simulink model "HydroPowertest"  (R2024b)
settings: Solver=FixedStepAuto  StartTime=0.0  StopTime=10  FixedStep=0.0001  RelTol=1e-3
values from neighbouring files (symbols this model uses):
  A = [0 Lq 0;-Ld 0 Mf]    [Generator_Datatest.m]
  Acc = [0 Lq 0;-Ld 0 Mf;0 0 0]    [Generator_Datatest.m]
  Af = 0.01    [Data__MOTOR.m]    (also in Generator_Data.m = 0.0001; Generator_Datatest.m)
  Bf = 0.0002    [Data__MOTOR.m]    (also in Generator_Data.m = 2e-05; Generator_Datatest.m)
  Cc = Cc0+6*Cc0    (= 0.7)    [Data__MOTOR.m]    (also in Generator_Datatest.m)
  Cc0 = 0.1    [Data__MOTOR.m]    (also in Generator_Datatest.m)
  CurrentFaultSwitch = 0    [Data__MOTOR.m]    (also in Generator_Data.m = 1; Generator_Datatest.m)
  Jm = 0.08    [Data__MOTOR.m]    (also in Generator_Datatest.m)
  Ke = 0.139    [Data__MOTOR.m]    (also in Generator_Datatest.m)
  Lcc = [-Ld 0 Mf;0 -Lq 0;-Mf 0 Lf]    [Generator_Datatest.m]
  Le = 0.44    [Data__MOTOR.m]    (also in Generator_Datatest.m)
  Lf = 0.0924    [Generator_Datatest.m]
  P = 4    [Generator_Data.m]    (also in Generator_Datatest.m = 3)
  R = 42.3    [Data__MOTOR.m]    (also in Generator_Datatest.m = [Rs 0 0;0 Rs 0])
  rate_noise_i = 0.02*In    (= 0.22)    [Data__MOTOR.m]    (also in Generator_Data.m = 0.02; Generator_Datatest.m)
  rate_noise_w = 0.02*Wn    (= 2.96)    [Data__MOTOR.m]    (also in Generator_Data.m = 0.002; Generator_Datatest.m)
  Rcc = [Rs 0 0;0 Rs 0;0 0 Rf]    [Generator_Datatest.m]
  Re = 2.4    [Data__MOTOR.m]    (also in Generator_Datatest.m)
  Rf = 10    [Generator_Datatest.m]
  Rm = 0.01    [Data__MOTOR.m]    (also in Generator_Datatest.m)
  sinamp = 384.6    [Generator_Datatest.m]
  StartStop = 0    [Data__MOTOR.m]    (also in Generator_Data.m; Generator_Datatest.m)
  Te = 0.1    [Data__MOTOR.m]    (also in Generator_Data.m = 1; Generator_Datatest.m)
  Ua = 48    [Data__MOTOR.m]    (also in Generator_Datatest.m)
  VelocityFaultSwitch = 0    [Data__MOTOR.m]    (also in Generator_Data.m = 1; Generator_Datatest.m)
  Vf = 300    [Generator_Datatest.m]
undefined symbols (not defined in the file or in its folder): dspblkCoreblockFVToolHelper, gcbh, sigbuilder_block
libraries: SignalEditorBlockLib x5
(part 1 of 3)
settings Model: Creator=belka  LastModifiedBy=Nasser
settings DebuggingCC: SignalResolutionControl=TryResolveAll
settings RTWCC: GPUComputeCapability=3.5

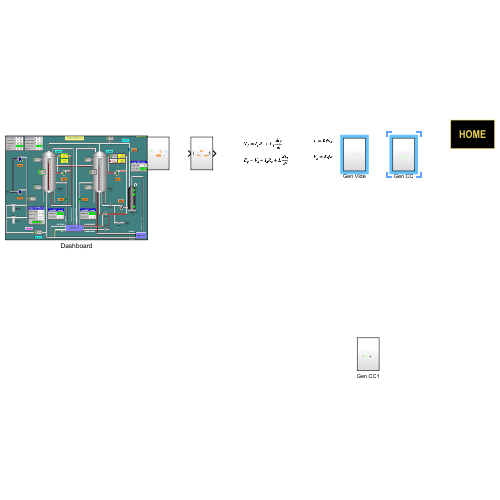
[thumbnail: Simulink's stored preview of the top-level diagram]
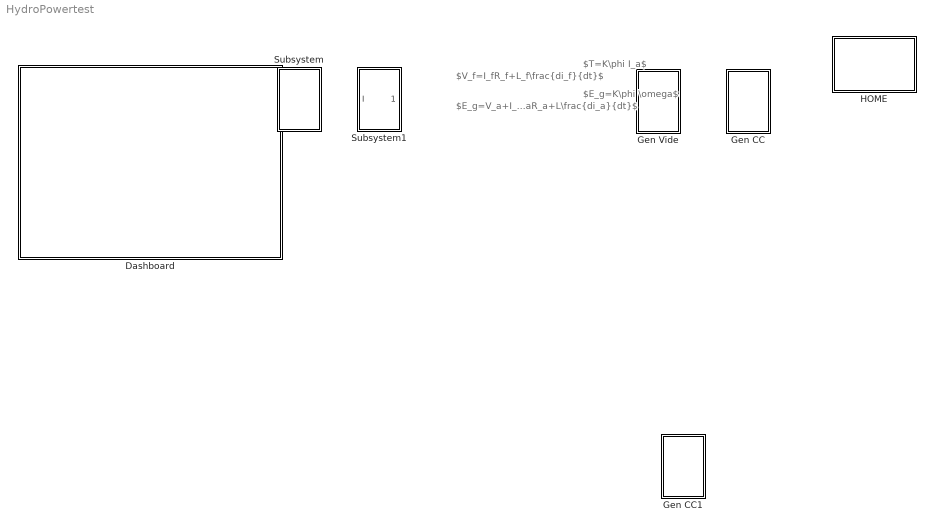
== system HydroPowertest ==
  note: $V_f=I_fR_f+L_f\frac{di_f}{dt}$
  note: $E_g=V_a+I_aR_a+L\frac{di_a}{dt}$
  note: $T=K\phi I_a$
  note: $E_g=K\phi \omega$
  Dashboard : Subsystem
      mask Display: image('scada.jpg');
  Gen CC : Subsystem
  Gen CC1 : Subsystem
  Gen Vide : Subsystem
  HOME : Subsystem
      settings: OpenFcn=MENU_SUPERVISION_MOTOR
      mask Display: disp('HOME')
  Subsystem : Subsystem
  Subsystem1 : Subsystem
